simulink model "RflyUdpUltraSimpleEight_Dist"  (R2022a)
settings: Solver=FixedStepDiscrete  StartTime=0.0  StopTime=inf  FixedStep=1/30  RelTol=1e-3  EnableMultiTasking=on
PreLoadFcn:
  | filepath  = fileparts(get_param(bdroot, 'FileName'))
  | cd(filepath);
undefined symbols (not defined in the file): Busy, Wait
libraries: aerolibanimutils x1
(part 1 of 2)
settings Model: Creator=dream  LastModifiedBy=23790
settings SolverCC: AlgebraicLoopSolver=TrustRegion
settings DataIOCC: SaveFormat=Array  SignalLoggingSaveFormat=ModelDataLogs  ReturnWorkspaceOutputs=off
settings OptimizationCC: BlockReduction=off  BooleanDataType=off  ZeroExternalMemoryAtStartup=off  ZeroInternalMemoryAtStartup=off
settings DebuggingCC: SaveWithParameterizedLinksMsg=none  UnderspecifiedInitializationDetection=Classic  MergeDetectMultiDrivingBlocksExec=none  SignalResolutionControl=TryResolveAllWithWarning  MultiTaskDSMMsg=warning  MultiTaskCondExecSysMsg=none  UnconnectedInputMsg=warning  UnconnectedOutputMsg=warning  UnconnectedLineMsg=warning  SFMachineParentedDataDiag=warning  ArithmeticOperatorsInVariantConditions=warning
settings HardwareCC: TargetBitPerPointer=64  TargetBitPerSizeT=64  TargetBitPerPtrDiffT=64  TargetLongLongMode=on  TargetIntDivRoundTo=Zero  TargetEndianess=LittleEndian  TargetWordSize=64  TargetHWDeviceType=MATLAB Host  ProdEqTarget=off
settings ModelReferenceCC: PropagateSignalLabelsOutOfModel=off
settings SFSimCC: SimUseLocalCustomCode=off  CustomCodeUndefinedFunction=UseInterfaceOnly  SimTargetLang=C++
settings RTWCC: PackageGeneratedCodeAndArtifacts=on  PackageName=RflyUdpExe  RTWUseLocalCustomCode=off  BuildConfiguration=Faster Runs  TargetLang=C++
settings GRTTargetCC: TargetLangStandard=C++03 (ISO)  CodeInterfacePackaging=C++ class  MultiInstanceErrorCode=None

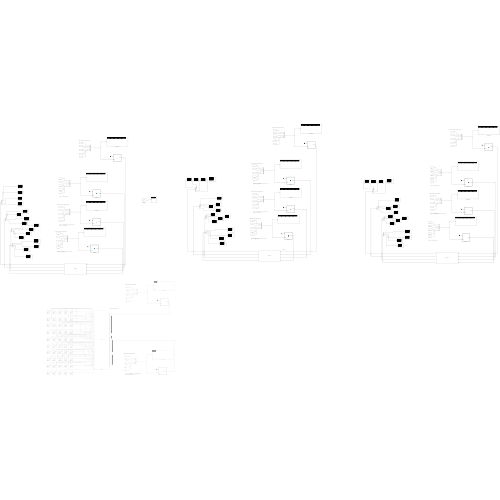
[thumbnail: Simulink's stored preview of the top-level diagram]
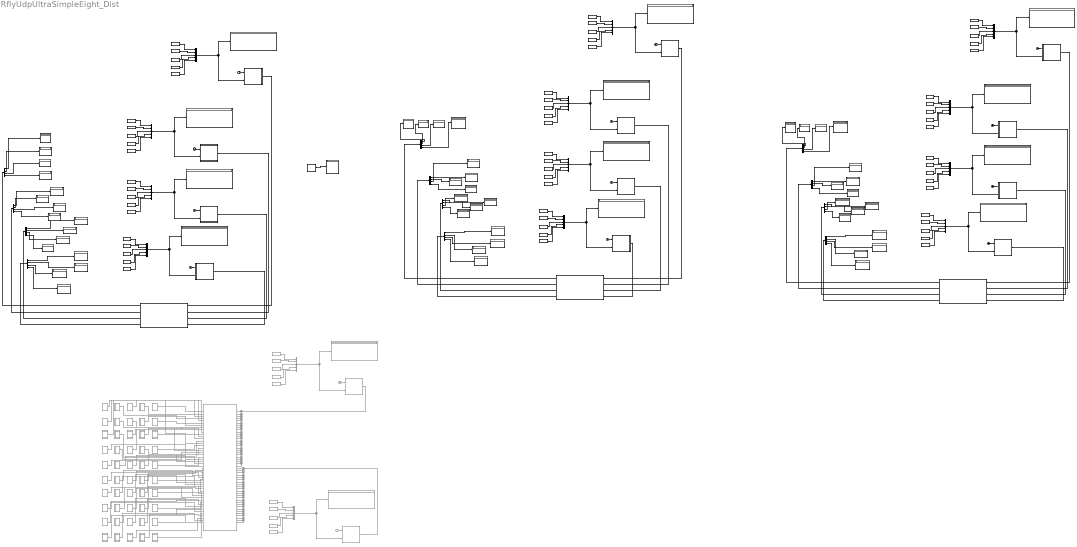
== system RflyUdpUltraSimpleEight_Dist ==
  note: 飞机状态反馈
  note: 0: Earth Vel; 1:Body Vel; 2: Earth Pos; 3:Body Pos
  note: 0: Earth Vel; 1:Body Vel; 2: Earth Pos; 3:Body Pos
  note: 这里展示了发送一条flag为2的消息，对应 地球坐标系下的位置指令
      | 发送本指令时，固定翼会飞到预设的点
  note: 这里展示了发送一条flag为2的消息，对应 地球坐标系下的位置指令
      | 发送本指令时，固定翼会飞到预设的点
  note: 0: Earth Vel; 1:Body Vel; 2: Earth Pos; 3:Body Pos
  note: 0: Earth Vel; 1:Body Vel; 2: Earth Pos; 3:Body Pos
  note: 这里展示了发送一条flag为2的消息，对应 地球坐标系下的位置指令
      | 发送本指令时，固定翼会飞到预设的点
  note: 这里展示了发送一条flag为2的消息，对应 地球坐标系下的位置指令
      | 发送本指令时，固定翼会飞到预设的点
  note: 0: Earth Vel; 1:Body Vel; 2: Earth Pos; 3:Body Pos
  note: 这里展示了发送一条flag为2的消息，对应 地球坐标系下的位置指令
      | 发送本指令时，固定翼会飞到预设的点
  note: 0: Earth Vel; 1:Body Vel; 2: Earth Pos; 3:Body Pos
  note: 0: Earth Vel; 1:Body Vel; 2: Earth Pos; 3:Body Pos
  note: 0: Earth Vel; 1:Body Vel; 2: Earth Pos; 3:Body Pos
  note: 这里展示了发送一条flag为2的消息，对应 地球坐标系下的位置指令
      | 发送本指令时，固定翼会飞到预设的点
  note: 这里展示了发送一条flag为2的消息，对应 地球坐标系下的位置指令
      | 发送本指令时，固定翼会飞到预设的点
  note: 0: Earth Vel; 1:Body Vel; 2: Earth Pos; 3:Body Pos
  note: 0: Earth Vel; 1:Body Vel; 2: Earth Pos; 3:Body Pos
  note: 这里展示了发送一条flag为2的消息，对应 地球坐标系下的位置指令
      | 发送本指令时，固定翼会飞到预设的点
  note: 飞机状态反馈
  note: 0: Earth Vel; 1:Body Vel; 2: Earth Pos; 3:Body Pos
  note: 这里展示了发送一条flag为2的消息，对应 地球坐标系下的位置指令
      | 发送本指令时，固定翼会飞到预设的点
  note: 这里展示了发送一条flag为2的消息，对应 地球坐标系下的位置指令
      | 发送本指令时，固定翼会飞到预设的点
  note: 0: Earth Vel; 1:Body Vel; 2: Earth Pos; 3:Body Pos
  note: 飞机状态反馈
  note: 0: Earth Vel; 1:Body Vel; 2: Earth Pos; 3:Body Pos
  note: 这里展示了发送一条flag为2的消息，对应 地球坐标系下的位置指令
      | 发送本指令时，固定翼会飞到预设的点
  note: 0: Earth Vel; 1:Body Vel; 2: Earth Pos; 3:Body Pos
  10号飞机状态反馈 : Subsystem  Commented=on
  10号飞机状态反馈1 : Subsystem  Commented=on
  10号飞机状态反馈2 : Subsystem  Commented=on
  10号飞机状态反馈3 : Subsystem  Commented=on
  10号飞机状态反馈4 : Subsystem  Commented=on
  1号飞机状态反馈 : Subsystem  Commented=on
  1号飞机状态反馈1 : Subsystem  Commented=on
  1号飞机状态反馈2 : Subsystem  Commented=on
  1号飞机状态反馈3 : Subsystem  Commented=on
  1号飞机状态反馈4 : Subsystem  Commented=on
  2号飞机状态反馈 : Subsystem  Commented=on
  2号飞机状态反馈1 : Subsystem  Commented=on
  2号飞机状态反馈2 : Subsystem  Commented=on
  2号飞机状态反馈3 : Subsystem  Commented=on
  2号飞机状态反馈4 : Subsystem  Commented=on
  3号飞机状态反馈 : Subsystem  Commented=on
  3号飞机状态反馈1 : Subsystem  Commented=on
  3号飞机状态反馈2 : Subsystem  Commented=on
  3号飞机状态反馈3 : Subsystem  Commented=on
  3号飞机状态反馈4 : Subsystem  Commented=on
  4号飞机状态反馈 : Subsystem  Commented=on
  4号飞机状态反馈1 : Subsystem  Commented=on
  4号飞机状态反馈2 : Subsystem  Commented=on
  4号飞机状态反馈3 : Subsystem  Commented=on
  4号飞机状态反馈4 : Subsystem  Commented=on
  5号飞机状态反馈 : Subsystem  Commented=on
  5号飞机状态反馈1 : Subsystem  Commented=on
  5号飞机状态反馈2 : Subsystem  Commented=on
  5号飞机状态反馈3 : Subsystem  Commented=on
  5号飞机状态反馈4 : Subsystem  Commented=on
  6号飞机状态反馈 : Subsystem  Commented=on
  6号飞机状态反馈1 : Subsystem  Commented=on
  6号飞机状态反馈2 : Subsystem  Commented=on
  6号飞机状态反馈3 : Subsystem  Commented=on
  6号飞机状态反馈4 : Subsystem  Commented=on
  7号飞机状态反馈 : Subsystem  Commented=on
  7号飞机状态反馈1 : Subsystem  Commented=on
  7号飞机状态反馈2 : Subsystem  Commented=on
  7号飞机状态反馈3 : Subsystem  Commented=on
  7号飞机状态反馈4 : Subsystem  Commented=on
  8号飞机状态反馈 : Subsystem  Commented=on
  8号飞机状态反馈1 : Subsystem  Commented=on
  8号飞机状态反馈2 : Subsystem  Commented=on
  8号飞机状态反馈3 : Subsystem  Commented=on
  8号飞机状态反馈4 : Subsystem  Commented=on
  9号飞机状态反馈 : Subsystem  Commented=on
  9号飞机状态反馈1 : Subsystem  Commented=on
  9号飞机状态反馈2 : Subsystem  Commented=on
  9号飞机状态反馈3 : Subsystem  Commented=on
  9号飞机状态反馈4 : Subsystem  Commented=on
  Clock : Clock  Commented=on
  Clock1 : Clock  Commented=on
  Clock{2..13} (12 alike) : Clock
  Commander : MATLAB Function  Commented=on  TreatAsAtomicUnit=on
  Commander1 : MATLAB Function  Commented=on  TreatAsAtomicUnit=on
  Commander10 : MATLAB Function  TreatAsAtomicUnit=on
  Commander11 : MATLAB Function  TreatAsAtomicUnit=on
  Commander12 : MATLAB Function  TreatAsAtomicUnit=on
  Commander13 : MATLAB Function  TreatAsAtomicUnit=on
  Commander2 : MATLAB Function  TreatAsAtomicUnit=on
  Commander3 : MATLAB Function  TreatAsAtomicUnit=on
  Commander4 : MATLAB Function  TreatAsAtomicUnit=on
  Commander5 : MATLAB Function  TreatAsAtomicUnit=on
  Commander6 : MATLAB Function  TreatAsAtomicUnit=on
  Commander7 : MATLAB Function  TreatAsAtomicUnit=on
  Commander8 : MATLAB Function  TreatAsAtomicUnit=on
  Commander9 : MATLAB Function  TreatAsAtomicUnit=on
  Demux{1..11,24} (12 alike) : Demux
  Display{,1..32,49..64} (49 alike) : Display
  Last Valid Data1 : Display  Commented=on
  Last Valid Data{2..3,5..14} (12 alike) : Display
  Last Valid Data4 : Display  Commented=on
  Mux{1..11,26} (12 alike) : Mux  Inputs=5
  Mux24 : Mux  Commented=on  Inputs=5
  Mux25 : Mux  Commented=on  Inputs=5
  PosX{,1..11} (12 alike) : Constant  Value=160
  PosX/Vel : Constant  Commented=on  Value=500
  PosX1/Vel1 : Constant  Commented=on  Value=500
  PosY{,1..11} (12 alike) : Constant  Value=-2000
  PosY/Alt : Constant  Commented=on  Value=-500
  PosY1/Yaw1 : Constant  Commented=on  Value=-500
  PosZ{,1..11} (12 alike) : Constant  Value=10/180*pi
  PosZ/Yaw : Constant  Commented=on
  PosZ1/Alt1 : Constant  Commented=on
  RflyUdpFast : S-Function  Commented=on  FunctionName=RflyUdpFast  Parameters=port,num,modeValue,T,ip  SFunctionDeploymentMode=off  EnableBusSupport=off  mask(UDP Receive){ip=192.168.31.11, port=20200, num=50, mode=UltraSimple Mode, T=1/30, modeValue=0}
      mask prompts: ip "UDP IP Address"; port "UDP Port"; num "vehicle Number"; mode "UDP Mode"; T "Sample Time"
      mask help:
      | This block receives bytes from an UDP/IP connection.
      | The first parameter is the UDP port on the first CopterSim App
      | The second parameter is the total vehicle number
      | The third parameter is the data mode. check the help button for the definition
      mask init:
      | if strcmp(mode,'FullData Mode')
      |     modeValue = 0;
      | elseif strcmp(mode,'SimpleData Mode') 
      |     modeValue = 1;
      | elseif strcmp(mode,'UltraSimple Mode') 
      |     modeValue = 2;
      | else
      |     modeValue = 0;
      | end
      mask Help:
      | UDP mode = 0 (localhost) or 1(broadcast), the 28-D output is defined as:
      | for(int i=0;i<3;i++){
      |     data[0+i]=(double)stl.gpsHome[i];
      |     data[3+i]=(double)stl.AngEular[i];
      |     data[6+i]=(double)stl.localPos[i];
      |     data[9+i]=(double)stl.localVel[i];
      |     data[12+i]=(double)stl.GpsPos[i];
      |     data[15+i]=(double)stl.GpsVel[i];
      | }
      | data[18] = (double)stl.time_boot_ms;
      | data[19] = (double)stl.copterID;
      | data[20] = (double)stl.relative_alt;
      | data[21] = (double)stl.hdg;
      | data[22] = (double)stl.satellites_visible;
      | data[23] = (double)stl.fix_type;
      | data[24] = (double)stl.resrveInit;
      | data[25] = (double)stl.pos_horiz_accuracy;
      | data[26] = (double)stl.pos_vert_accuracy;
      | data[27] = (double)stl.resrveFloat;
      | 
      | UDP mode =  2 (localhost) or 3(broadcast), 4,5 the 12-D output is defined as:
      | 
      | if(iUdpMode==2||iUdpMode==3){
      |     for(int i=0;i<3;i++){
      |         data[i]=(double)st.gpsHome[i];
      |         data[i+3]=(double)st.AngEular[i];
      |         data[i+6]=(double)st.localPos[i];
      |         data[i+9]=(double)st.localVel[i];
      |     }
      | }
      | if(iUdpMode==4||iUdpMode==5){
      |     double GpsHomePos[3];
      |     for(int i=0;i<3;i++){
      |             GpsHomePos[i] = (double)st.gpsHome[i];
      |             data[3+i]=(double)st.localPos[i];
      |             data[6+i]=(double)st.localVel[i];
      |             data[9+i]=(double)st.AngEular[i];
      |     }
      |     double PIR = 3.1415926536;
      |     data[0]=(GpsHomePos[0]*1e-7-40.1540302)/180*PIR*6362000+(double)st.localPos[0];
      |     data[1]=(GpsHomePos[1]*1e-7-116.2593683)/180*PIR*6362000+(double)st.localPos[1];
      |     data[2]=-GpsHomePos[2]*1e-3+(double)st.localPos[2];
      | }
      | 
      | The above structure is
      | struct outHILStateData{ // mavlink data forward from Pixhawk
      |     uint32_t time_boot_ms; //Timestamp of the message
      |     uint32_t copterID;     //Copter ID start from 1
      |     int32_t GpsPos[3];     //Estimated GPS position，lat&long: deg*1e7, alt: m*1e3 and up is positive
      |     int32_t GpsVel[3];     //Estimated GPS velocity, NED, m/s*1e2->cm/s
      |     int32_t gpsHome[3];     //Home GPS position, lat&long: deg*1e7, alt: m*1e3 and up is positive
      |     int32_t relative_alt;  //alt: m*1e3 and up is positive
      |     int32_t hdg;           //Course angle, NED,deg*1000, 0~360
      |     int32_t satellites_visible; //GPS Raw data, sum of satellite
      |     int32_t fix_type;     //GPS Raw data, Fixed type, 3 for fixed (good precision)
      |     int32_t resrveInit;       //Int, reserve for the future use
      |     float AngEular[3];    //Estimated Euler angle, unit: rad/s
      |     float localPos[3];    //Estimated locoal position, NED, unit: m
      |     float localVel[3];    //Estimated locoal velocity, NED, unit: m/s
      |     float pos_horiz_accuracy;   //GPS horizontal accuracy, unit: m
      |     float pos_vert_accuracy; //GPS vertical accuracy, unit: m
      |     float resrveFloat;      //float,reserve for the future use
      | }
      mask TypeOptions mode: FullData Mode | SimpleData Mode | UltraSimple Mode
  Simulation Pace1 : aerolibanimutils/Simulation Pace  SimulationPace=1  SleepMode=Busy-Wait  OutputPaceError=on  SampleTime=-1
  UDP Recv1 : S-Function  FunctionName=RflyUdpFast  Parameters=port,num,modeValue,T,ip  SFunctionDeploymentMode=off  EnableBusSupport=off  mask(UDP Receive){ip=192.168.31.253, port=20100, num=4, mode=UltraSimple Mode, T=1/30, modeValue=0}
      mask prompts: ip "UDP IP Address"; port "UDP Port"; num "vehicle Number"; mode "UDP Mode"; T "Sample Time"
      mask help:
      | This block receives bytes from an UDP/IP connection.
      | The first parameter is the UDP port on the first CopterSim App
      | The second parameter is the total vehicle number
      | The third parameter is the data mode. check the help button for the definition
      mask init:
      | if strcmp(mode,'FullData Mode')
      |     modeValue = 0;
      | elseif strcmp(mode,'SimpleData Mode') 
      |     modeValue = 1;
      | elseif strcmp(mode,'UltraSimple Mode') 
      |     modeValue = 2;
      | else
      |     modeValue = 0;
      | end
      mask Help:
      | UDP mode = 0 (localhost) or 1(broadcast), the 28-D output is defined as:
      | for(int i=0;i<3;i++){
      |     data[0+i]=(double)stl.gpsHome[i];
      |     data[3+i]=(double)stl.AngEular[i];
      |     data[6+i]=(double)stl.localPos[i];
      |     data[9+i]=(double)stl.localVel[i];
      |     data[12+i]=(double)stl.GpsPos[i];
      |     data[15+i]=(double)stl.GpsVel[i];
      | }
      | data[18] = (double)stl.time_boot_ms;
      | data[19] = (double)stl.copterID;
      | data[20] = (double)stl.relative_alt;
      | data[21] = (double)stl.hdg;
      | data[22] = (double)stl.satellites_visible;
      | data[23] = (double)stl.fix_type;
      | data[24] = (double)stl.resrveInit;
      | data[25] = (double)stl.pos_horiz_accuracy;
      | data[26] = (double)stl.pos_vert_accuracy;
      | data[27] = (double)stl.resrveFloat;
      | 
      | UDP mode =  2 (localhost) or 3(broadcast), 4,5 the 12-D output is defined as:
      | 
      | if(iUdpMode==2||iUdpMode==3){
      |     for(int i=0;i<3;i++){
      |         data[i]=(double)st.gpsHome[i];
      |         data[i+3]=(double)st.AngEular[i];
      |         data[i+6]=(double)st.localPos[i];
      |         data[i+9]=(double)st.localVel[i];
      |     }
      | }
      | if(iUdpMode==4||iUdpMode==5){
      |     double GpsHomePos[3];
      |     for(int i=0;i<3;i++){
      |             GpsHomePos[i] = (double)st.gpsHome[i];
      |             data[3+i]=(double)st.localPos[i];
      |             data[6+i]=(double)st.localVel[i];
      |             data[9+i]=(double)st.AngEular[i];
      |     }
      |     double PIR = 3.1415926536;
      |     data[0]=(GpsHomePos[0]*1e-7-40.1540302)/180*PIR*6362000+(double)st.localPos[0];
      |     data[1]=(GpsHomePos[1]*1e-7-116.2593683)/180*PIR*6362000+(double)st.localPos[1];
      |     data[2]=-GpsHomePos[2]*1e-3+(double)st.localPos[2];
      | }
      | 
      | The above structure is
      | struct outHILStateData{ // mavlink data forward from Pixhawk
      |     uint32_t time_boot_ms; //Timestamp of the message
      |     uint32_t copterID;     //Copter ID start from 1
      |     int32_t GpsPos[3];     //Estimated GPS position，lat&long: deg*1e7, alt: m*1e3 and up is positive
      |     int32_t GpsVel[3];     //Estimated GPS velocity, NED, m/s*1e2->cm/s
      |     int32_t gpsHome[3];     //Home GPS position, lat&long: deg*1e7, alt: m*1e3 and up is positive
      |     int32_t relative_alt;  //alt: m*1e3 and up is positive
      |     int32_t hdg;           //Course angle, NED,deg*1000, 0~360
      |     int32_t satellites_visible; //GPS Raw data, sum of satellite
      |     int32_t fix_type;     //GPS Raw data, Fixed type, 3 for fixed (good precision)
      |     int32_t resrveInit;       //Int, reserve for the future use
      |     float AngEular[3];    //Estimated Euler angle, unit: rad/s
      |     float localPos[3];    //Estimated locoal position, NED, unit: m
      |     float localVel[3];    //Estimated locoal velocity, NED, unit: m/s
      |     float pos_horiz_accuracy;   //GPS horizontal accuracy, unit: m
      |     float pos_vert_accuracy; //GPS vertical accuracy, unit: m
      |     float resrveFloat;      //float,reserve for the future use
      | }
      mask TypeOptions mode: FullData Mode | SimpleData Mode | UltraSimple Mode
  UDP Recv2 : S-Function  FunctionName=RflyUdpFast  Parameters=port,num,modeValue,T,ip  SFunctionDeploymentMode=off  EnableBusSupport=off  mask(UDP Receive){ip=192.168.31.15, port=20116, num=4, mode=UltraSimple Mode, T=1/30, modeValue=0}
      mask prompts: ip "UDP IP Address"; port "UDP Port"; num "vehicle Number"; mode "UDP Mode"; T "Sample Time"
      mask help:
      | This block receives bytes from an UDP/IP connection.
      | The first parameter is the UDP port on the first CopterSim App
      | The second parameter is the total vehicle number
      | The third parameter is the data mode. check the help button for the definition
      mask init:
      | if strcmp(mode,'FullData Mode')
      |     modeValue = 0;
      | elseif strcmp(mode,'SimpleData Mode') 
      |     modeValue = 1;
      | elseif strcmp(mode,'UltraSimple Mode') 
      |     modeValue = 2;
      | else
      |     modeValue = 0;
      | end
      mask Help:
      | UDP mode = 0 (localhost) or 1(broadcast), the 28-D output is defined as:
      | for(int i=0;i<3;i++){
      |     data[0+i]=(double)stl.gpsHome[i];
      |     data[3+i]=(double)stl.AngEular[i];
      |     data[6+i]=(double)stl.localPos[i];
      |     data[9+i]=(double)stl.localVel[i];
      |     data[12+i]=(double)stl.GpsPos[i];
      |     data[15+i]=(double)stl.GpsVel[i];
      | }
      | data[18] = (double)stl.time_boot_ms;
      | data[19] = (double)stl.copterID;
      | data[20] = (double)stl.relative_alt;
      | data[21] = (double)stl.hdg;
      | data[22] = (double)stl.satellites_visible;
      | data[23] = (double)stl.fix_type;
      | data[24] = (double)stl.resrveInit;
      | data[25] = (double)stl.pos_horiz_accuracy;
      | data[26] = (double)stl.pos_vert_accuracy;
      | data[27] = (double)stl.resrveFloat;
      | 
      | UDP mode =  2 (localhost) or 3(broadcast), 4,5 the 12-D output is defined as:
      | 
      | if(iUdpMode==2||iUdpMode==3){
      |     for(int i=0;i<3;i++){
      |         data[i]=(double)st.gpsHome[i];
      |         data[i+3]=(double)st.AngEular[i];
      |         data[i+6]=(double)st.localPos[i];
      |         data[i+9]=(double)st.localVel[i];
      |     }
      | }
      | if(iUdpMode==4||iUdpMode==5){
      |     double GpsHomePos[3];
      |     for(int i=0;i<3;i++){
      |             GpsHomePos[i] = (double)st.gpsHome[i];
      |             data[3+i]=(double)st.localPos[i];
      |             data[6+i]=(double)st.localVel[i];
      |             data[9+i]=(double)st.AngEular[i];
      |     }
      |     double PIR = 3.1415926536;
      |     data[0]=(GpsHomePos[0]*1e-7-40.1540302)/180*PIR*6362000+(double)st.localPos[0];
      |     data[1]=(GpsHomePos[1]*1e-7-116.2593683)/180*PIR*6362000+(double)st.localPos[1];
      |     data[2]=-GpsHomePos[2]*1e-3+(double)st.localPos[2];
      | }
      | 
      | The above structure is
      | struct outHILStateData{ // mavlink data forward from Pixhawk
      |     uint32_t time_boot_ms; //Timestamp of the message
      |     uint32_t copterID;     //Copter ID start from 1
      |     int32_t GpsPos[3];     //Estimated GPS position，lat&long: deg*1e7, alt: m*1e3 and up is positive
      |     int32_t GpsVel[3];     //Estimated GPS velocity, NED, m/s*1e2->cm/s
      |     int32_t gpsHome[3];     //Home GPS position, lat&long: deg*1e7, alt: m*1e3 and up is positive
      |     int32_t relative_alt;  //alt: m*1e3 and up is positive
      |     int32_t hdg;           //Course angle, NED,deg*1000, 0~360
      |     int32_t satellites_visible; //GPS Raw data, sum of satellite
      |     int32_t fix_type;     //GPS Raw data, Fixed type, 3 for fixed (good precision)
      |     int32_t resrveInit;       //Int, reserve for the future use
      |     float AngEular[3];    //Estimated Euler angle, unit: rad/s
      |     float localPos[3];    //Estimated locoal position, NED, unit: m
      |     float localVel[3];    //Estimated locoal velocity, NED, unit: m/s
      |     float pos_horiz_accuracy;   //GPS horizontal accuracy, unit: m
      |     float pos_vert_accuracy; //GPS vertical accuracy, unit: m
      |     float resrveFloat;      //float,reserve for the future use
      | }
      mask TypeOptions mode: FullData Mode | SimpleData Mode | UltraSimple Mode
  UDP Recv4 : S-Function  FunctionName=RflyUdpFast  Parameters=port,num,modeValue,T,ip  SFunctionDeploymentMode=off  EnableBusSupport=off  mask(UDP Receive){ip=192.168.31.13, port=20108, num=4, mode=UltraSimple Mode, T=1/30, modeValue=0}
      mask prompts: ip "UDP IP Address"; port "UDP Port"; num "vehicle Number"; mode "UDP Mode"; T "Sample Time"
      mask help:
      | This block receives bytes from an UDP/IP connection.
      | The first parameter is the UDP port on the first CopterSim App
      | The second parameter is the total vehicle number
      | The third parameter is the data mode. check the help button for the definition
      mask init:
      | if strcmp(mode,'FullData Mode')
      |     modeValue = 0;
      | elseif strcmp(mode,'SimpleData Mode') 
      |     modeValue = 1;
      | elseif strcmp(mode,'UltraSimple Mode') 
      |     modeValue = 2;
      | else
      |     modeValue = 0;
      | end
      mask Help:
      | UDP mode = 0 (localhost) or 1(broadcast), the 28-D output is defined as:
      | for(int i=0;i<3;i++){
      |     data[0+i]=(double)stl.gpsHome[i];
      |     data[3+i]=(double)stl.AngEular[i];
      |     data[6+i]=(double)stl.localPos[i];
      |     data[9+i]=(double)stl.localVel[i];
      |     data[12+i]=(double)stl.GpsPos[i];
      |     data[15+i]=(double)stl.GpsVel[i];
      | }
      | data[18] = (double)stl.time_boot_ms;
      | data[19] = (double)stl.copterID;
      | data[20] = (double)stl.relative_alt;
      | data[21] = (double)stl.hdg;
      | data[22] = (double)stl.satellites_visible;
      | data[23] = (double)stl.fix_type;
      | data[24] = (double)stl.resrveInit;
      | data[25] = (double)stl.pos_horiz_accuracy;
      | data[26] = (double)stl.pos_vert_accuracy;
      | data[27] = (double)stl.resrveFloat;
      | 
      | UDP mode =  2 (localhost) or 3(broadcast), 4,5 the 12-D output is defined as:
      | 
      | if(iUdpMode==2||iUdpMode==3){
      |     for(int i=0;i<3;i++){
      |         data[i]=(double)st.gpsHome[i];
      |         data[i+3]=(double)st.AngEular[i];
      |         data[i+6]=(double)st.localPos[i];
      |         data[i+9]=(double)st.localVel[i];
      |     }
      | }
      | if(iUdpMode==4||iUdpMode==5){
      |     double GpsHomePos[3];
      |     for(int i=0;i<3;i++){
      |             GpsHomePos[i] = (double)st.gpsHome[i];
      |             data[3+i]=(double)st.localPos[i];
      |             data[6+i]=(double)st.localVel[i];
      |             data[9+i]=(double)st.AngEular[i];
      |     }
      |     double PIR = 3.1415926536;
      |     data[0]=(GpsHomePos[0]*1e-7-40.1540302)/180*PIR*6362000+(double)st.localPos[0];
      |     data[1]=(GpsHomePos[1]*1e-7-116.2593683)/180*PIR*6362000+(double)st.localPos[1];
      |     data[2]=-GpsHomePos[2]*1e-3+(double)st.localPos[2];
      | }
      | 
      | The above structure is
      | struct outHILStateData{ // mavlink data forward from Pixhawk
      |     uint32_t time_boot_ms; //Timestamp of the message
      |     uint32_t copterID;     //Copter ID start from 1
      |     int32_t GpsPos[3];     //Estimated GPS position，lat&long: deg*1e7, alt: m*1e3 and up is positive
      |     int32_t GpsVel[3];     //Estimated GPS velocity, NED, m/s*1e2->cm/s
      |     int32_t gpsHome[3];     //Home GPS position, lat&long: deg*1e7, alt: m*1e3 and up is positive
      |     int32_t relative_alt;  //alt: m*1e3 and up is positive
      |     int32_t hdg;           //Course angle, NED,deg*1000, 0~360
      |     int32_t satellites_visible; //GPS Raw data, sum of satellite
      |     int32_t fix_type;     //GPS Raw data, Fixed type, 3 for fixed (good precision)
      |     int32_t resrveInit;       //Int, reserve for the future use
      |     float AngEular[3];    //Estimated Euler angle, unit: rad/s
      |     float localPos[3];    //Estimated locoal position, NED, unit: m
      |     float localVel[3];    //Estimated locoal velocity, NED, unit: m/s
      |     float pos_horiz_accuracy;   //GPS horizontal accuracy, unit: m
      |     float pos_vert_accuracy; //GPS vertical accuracy, unit: m
      |     float resrveFloat;      //float,reserve for the future use
      | }
      mask TypeOptions mode: FullData Mode | SimpleData Mode | UltraSimple Mode
  flag : Constant  Commented=on  Value=13
  flag1 : Constant  Commented=on  Value=13
  flag{2..13} (12 alike) : Constant  Value=13
  yaw : Constant  Commented=on  Value=0
  yaw1 : Constant  Commented=on  Value=0
  yaw{2..13} (12 alike) : Constant  Value=0
  wires:
  UDP Recv1/1 -> Demux4/1
  Simulation Pace1/1 -> Display/1
  Demux4/1 -> Display1/1
  Demux4/3 -> Display3/1
  Demux4/4 -> Display4/1
  Demux5/4 -> Display8/1
  Demux5/3 -> Display7/1
  Demux5/1 -> Display5/1
  Demux6/4 -> Display12/1
  Demux6/3 -> Display11/1
  Demux6/1 -> Display9/1
  UDP Recv1/2 -> Demux5/1
  UDP Recv1/3 -> Demux6/1
  Demux4/2 -> Display2/1
  Demux5/2 -> Display6/1
  Demux6/2 -> Display10/1
  Demux7/2 -> Display14/1
  Demux7/4 -> Display16/1
  UDP Recv1/4 -> Demux7/1
  Demux7/1 -> Display13/1
  Demux7/3 -> Display15/1
  RflyUdpFast/44 -> 4号飞机状态反馈4/1(In1)
  RflyUdpFast/9 -> 9号飞机状态反馈/1(In1)
  RflyUdpFast/48 -> 8号飞机状态反馈4/1(In1)
  Commander/1(outCMDs) -> RflyUdpFast/5, RflyUdpFast/6, RflyUdpFast/7, RflyUdpFast/8, RflyUdpFast/9, RflyUdpFast/10, RflyUdpFast/11, RflyUdpFast/12, RflyUdpFast/13, RflyUdpFast/14, RflyUdpFast/15, RflyUdpFast/16, RflyUdpFast/17, RflyUdpFast/18, RflyUdpFast/19, RflyUdpFast/20, RflyUdpFast/21, RflyUdpFast/22, RflyUdpFast/23, RflyUdpFast/24, RflyUdpFast/25, RflyUdpFast/4, RflyUdpFast/3, RflyUdpFast/2, RflyUdpFast/1
  RflyUdpFast/22 -> 2号飞机状态反馈2/1(In1)
  RflyUdpFast/27 -> 7号飞机状态反馈2/1(In1)
  RflyUdpFast/49 -> 9号飞机状态反馈4/1(In1)
  RflyUdpFast/40 -> 10号飞机状态反馈3/1(In1)
  RflyUdpFast/45 -> 5号飞机状态反馈4/1(In1)
  RflyUdpFast/18 -> 8号飞机状态反馈1/1(In1)
  RflyUdpFast/37 -> 7号飞机状态反馈3/1(In1)
  RflyUdpFast/25 -> 5号飞机状态反馈2/1(In1)
  Commander1/1(outCMDs) -> RflyUdpFast/50, RflyUdpFast/49, RflyUdpFast/48, RflyUdpFast/47, RflyUdpFast/46, RflyUdpFast/45, RflyUdpFast/44, RflyUdpFast/43, RflyUdpFast/42, RflyUdpFast/41, RflyUdpFast/40, RflyUdpFast/39, RflyUdpFast/38, RflyUdpFast/37, RflyUdpFast/36, RflyUdpFast/35, RflyUdpFast/34, RflyUdpFast/33, RflyUdpFast/32, RflyUdpFast/31, RflyUdpFast/30, RflyUdpFast/29, RflyUdpFast/28, RflyUdpFast/27, RflyUdpFast/26
  RflyUdpFast/7 -> 7号飞机状态反馈/1(In1)
  RflyUdpFast/50 -> 10号飞机状态反馈4/1(In1)
  RflyUdpFast/42 -> 2号飞机状态反馈4/1(In1)
  RflyUdpFast/3 -> 3号飞机状态反馈/1(In1)
  RflyUdpFast/39 -> 9号飞机状态反馈3/1(In1)
  yaw/1 -> Mux24/5
  RflyUdpFast/21 -> 1号飞机状态反馈2/1(In1)
  RflyUdpFast/35 -> 5号飞机状态反馈3/1(In1)
  RflyUdpFast/6 -> 6号飞机状态反馈/1(In1)
  RflyUdpFast/33 -> 3号飞机状态反馈3/1(In1)
  RflyUdpFast/34 -> 4号飞机状态反馈3/1(In1)
  RflyUdpFast/24 -> 4号飞机状态反馈2/1(In1)
  RflyUdpFast/11 -> 1号飞机状态反馈1/1(In1)
  RflyUdpFast/12 -> 2号飞机状态反馈1/1(In1)
  flag/1 -> Mux24/1
  RflyUdpFast/23 -> 3号飞机状态反馈2/1(In1)
  PosY/Alt/1 -> Mux24/3
  RflyUdpFast/47 -> 7号飞机状态反馈4/1(In1)
  RflyUdpFast/31 -> 1号飞机状态反馈3/1(In1)
  Clock1/1 -> Commander1/1(t)
  RflyUdpFast/8 -> 8号飞机状态反馈/1(In1)
  RflyUdpFast/43 -> 3号飞机状态反馈4/1(In1)
  RflyUdpFast/16 -> 6号飞机状态反馈1/1(In1)
  RflyUdpFast/29 -> 9号飞机状态反馈2/1(In1)
  RflyUdpFast/30 -> 10号飞机状态反馈2/1(In1)
  Mux25/1 -> Last Valid Data1/1, Commander1/2(inCMDs)
  Clock/1 -> Commander/1(t)
  PosX/Vel/1 -> Mux24/2
  RflyUdpFast/20 -> 10号飞机状态反馈1/1(In1)
  RflyUdpFast/19 -> 9号飞机状态反馈1/1(In1)
  RflyUdpFast/15 -> 5号飞机状态反馈1/1(In1)
  RflyUdpFast/26 -> 6号飞机状态反馈2/1(In1)
  PosY1/Yaw1/1 -> Mux25/3
  RflyUdpFast/4 -> 4号飞机状态反馈/1(In1)
  RflyUdpFast/36 -> 6号飞机状态反馈3/1(In1)
  PosZ/Yaw/1 -> Mux24/4
  RflyUdpFast/17 -> 7号飞机状态反馈1/1(In1)
  PosX1/Vel1/1 -> Mux25/2
  RflyUdpFast/5 -> 5号飞机状态反馈/1(In1)
  RflyUdpFast/38 -> 8号飞机状态反馈3/1(In1)
  yaw1/1 -> Mux25/5
  RflyUdpFast/10 -> 10号飞机状态反馈/1(In1)
  RflyUdpFast/46 -> 6号飞机状态反馈4/1(In1)
  RflyUdpFast/41 -> 1号飞机状态反馈4/1(In1)
  RflyUdpFast/13 -> 3号飞机状态反馈1/1(In1)
  RflyUdpFast/1 -> 1号飞机状态反馈/1(In1)
  RflyUdpFast/32 -> 2号飞机状态反馈3/1(In1)
  RflyUdpFast/14 -> 4号飞机状态反馈1/1(In1)
  flag1/1 -> Mux25/1
  RflyUdpFast/2 -> 2号飞机状态反馈/1(In1)
  RflyUdpFast/28 -> 8号飞机状态反馈2/1(In1)
  Mux24/1 -> Last Valid Data4/1, Commander/2(inCMDs)
  PosZ1/Alt1/1 -> Mux25/4
  yaw2/1 -> Mux26/5
  Mux26/1 -> Last Valid Data2/1, Commander2/2(inCMDs)
  PosY/1 -> Mux26/3
  Clock2/1 -> Commander2/1(t)
  flag2/1 -> Mux26/1
  PosZ/1 -> Mux26/4
  PosX/1 -> Mux26/2
  Commander2/1(outCMDs) -> UDP Recv1/1
  Clock3/1 -> Commander3/1(t)
  yaw3/1 -> Mux2/5
  PosX1/1 -> Mux2/2
  flag3/1 -> Mux2/1
  Commander3/1(outCMDs) -> UDP Recv1/2
  PosY1/1 -> Mux2/3
  Mux2/1 -> Last Valid Data3/1, Commander3/2(inCMDs)
  PosZ1/1 -> Mux2/4
  PosX2/1 -> Mux3/2
  PosY2/1 -> Mux3/3
  Commander4/1(outCMDs) -> UDP Recv1/3
  flag4/1 -> Mux3/1
  Mux3/1 -> Commander4/2(inCMDs), Last Valid Data5/1
  yaw4/1 -> Mux3/5
  Clock4/1 -> Commander4/1(t)
  PosZ2/1 -> Mux3/4
  PosY3/1 -> Mux4/3
  Clock5/1 -> Commander5/1(t)
  PosZ3/1 -> Mux4/4
  Mux4/1 -> Last Valid Data6/1, Commander5/2(inCMDs)
  Commander5/1(outCMDs) -> UDP Recv1/4
  yaw5/1 -> Mux4/5
  flag5/1 -> Mux4/1
  PosX3/1 -> Mux4/2
  Commander9/1(outCMDs) -> UDP Recv4/4
  PosX7/1 -> Mux7/2
  PosZ5/1 -> Mux1/4
  PosY5/1 -> Mux1/3
  Mux1/1 -> Last Valid Data8/1, Commander7/2(inCMDs)
  PosX5/1 -> Mux1/2
  Clock9/1 -> Commander9/1(t)
  PosY4/1 -> Mux5/3
  Commander6/1(outCMDs) -> UDP Recv4/1
  PosZ4/1 -> Mux5/4
  flag6/1 -> Mux5/1
  Commander8/1(outCMDs) -> UDP Recv4/3
  PosX4/1 -> Mux5/2
  yaw8/1 -> Mux6/5
  Clock6/1 -> Commander6/1(t)
  PosY6/1 -> Mux6/3
  PosX6/1 -> Mux6/2
  flag8/1 -> Mux6/1
  Demux24/3 -> Display55/1
  yaw6/1 -> Mux5/5
  UDP Recv4/3 -> Demux3/1
  Clock7/1 -> Commander7/1(t)
  yaw7/1 -> Mux1/5
  Demux3/2 -> Display50/1
  Demux3/3 -> Display51/1
  Clock8/1 -> Commander8/1(t)
  Demux24/4 -> Display56/1
  UDP Recv4/4 -> Demux24/1
  Demux2/1 -> Display60/1
  Demux2/3 -> Display62/1
  Demux24/1 -> Display53/1
  Mux5/1 -> Last Valid Data7/1, Commander6/2(inCMDs)
  Demux3/4 -> Display52/1
  Demux2/4 -> Display63/1
  Demux3/1 -> Display64/1
  PosY7/1 -> Mux7/3
  Demux1/1 -> Display49/1
  Demux1/3 -> Display58/1
  Mux6/1 -> Commander8/2(inCMDs), Last Valid Data9/1
  PosZ6/1 -> Mux6/4
  UDP Recv4/2 -> Demux2/1
  Demux1/4 -> Display59/1
  Demux2/2 -> Display61/1
  Mux7/1 -> Last Valid Data10/1, Commander9/2(inCMDs)
  PosZ7/1 -> Mux7/4
  Commander7/1(outCMDs) -> UDP Recv4/2
  flag9/1 -> Mux7/1
  Demux24/2 -> Display54/1
  yaw9/1 -> Mux7/5
  Demux1/2 -> Display57/1
  UDP Recv4/1 -> Demux1/1
  flag7/1 -> Mux1/1
  PosZ8/1 -> Mux9/4
  PosX8/1 -> Mux9/2
  yaw12/1 -> Mux10/5
  flag10/1 -> Mux9/1
  Commander10/1(outCMDs) -> UDP Recv2/1
  Mux8/1 -> Last Valid Data13/1, Commander11/2(inCMDs)
  PosX9/1 -> Mux8/2
  Clock13/1 -> Commander13/1(t)
  PosY9/1 -> Mux8/3
  Commander13/1(outCMDs) -> UDP Recv2/4
  Mux10/1 -> Commander12/2(inCMDs), Last Valid Data14/1
  PosY11/1 -> Mux11/3
  PosX11/1 -> Mux11/2
  Demux9/4 -> Display31/1
  Demux10/1 -> Display21/1
  Demux9/1 -> Display28/1
  UDP Recv2/4 -> Demux10/1
  Demux10/4 -> Display24/1
  Demux8/1 -> Display17/1
  Clock12/1 -> Commander12/1(t)
  yaw10/1 -> Mux9/5
  PosZ10/1 -> Mux10/4
  Demux10/3 -> Display23/1
  yaw11/1 -> Mux8/5
  Clock10/1 -> Commander10/1(t)
  Demux11/2 -> Display18/1
  Clock11/1 -> Commander11/1(t)
  Demux11/1 -> Display32/1
  PosX10/1 -> Mux10/2
  UDP Recv2/2 -> Demux9/1
  Demux8/4 -> Display27/1
  Mux9/1 -> Last Valid Data12/1, Commander10/2(inCMDs)
  UDP Recv2/1 -> Demux8/1
  flag12/1 -> Mux10/1
  flag13/1 -> Mux11/1
  PosZ9/1 -> Mux8/4
  Mux11/1 -> Last Valid Data11/1, Commander13/2(inCMDs)
  Demux8/3 -> Display26/1
  PosY8/1 -> Mux9/3
  Demux9/2 -> Display29/1
  Demux11/3 -> Display19/1
  yaw13/1 -> Mux11/5
  PosY10/1 -> Mux10/3
  Demux11/4 -> Display20/1
  Commander11/1(outCMDs) -> UDP Recv2/2
  Demux10/2 -> Display22/1
  flag11/1 -> Mux8/1
  Demux9/3 -> Display30/1
  Demux8/2 -> Display25/1
  PosZ11/1 -> Mux11/4
  UDP Recv2/3 -> Demux11/1
  Commander12/1(outCMDs) -> UDP Recv2/3

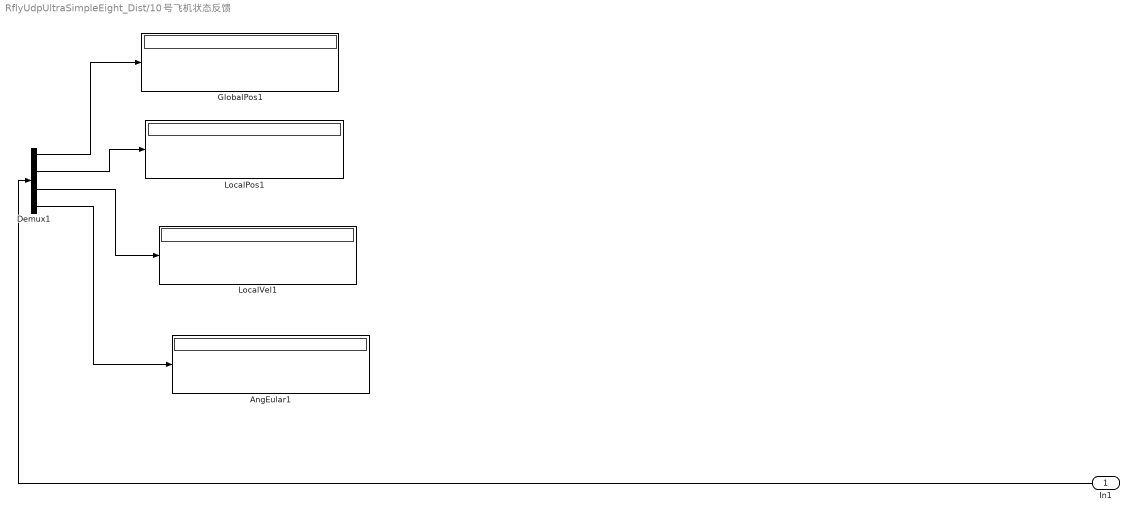
== system RflyUdpUltraSimpleEight_Dist/10号飞机状态反馈 ==
  In1 : Inport
  AngEular1 : Display
  Demux1 : Demux
  GlobalPos1 : Display
  LocalPos1 : Display
  LocalVel1 : Display
  wires:
  Demux1/2 -> LocalPos1/1
  Demux1/3 -> LocalVel1/1
  In1/1 -> Demux1/1
  Demux1/1 -> GlobalPos1/1
  Demux1/4 -> AngEular1/1

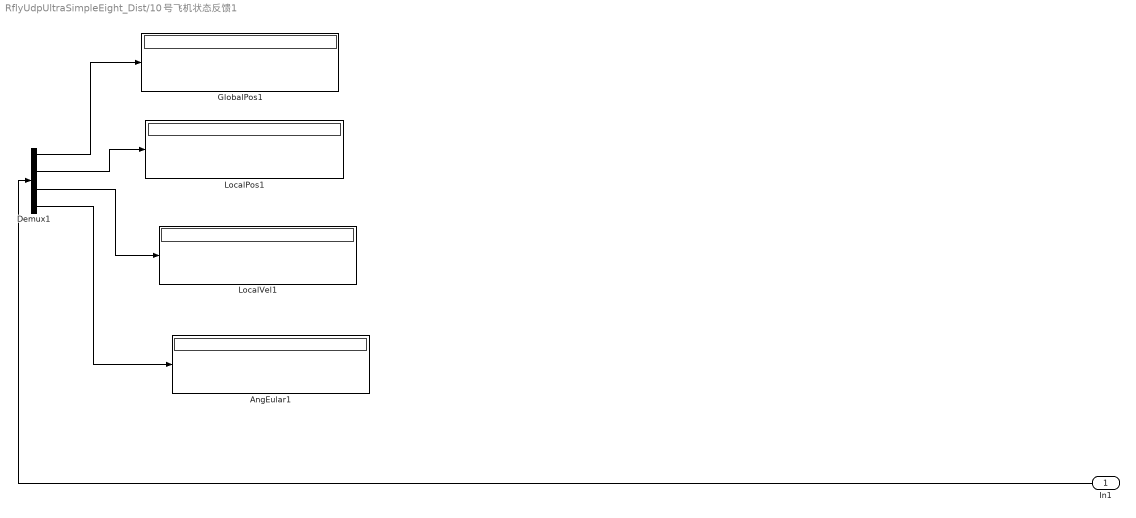
== system RflyUdpUltraSimpleEight_Dist/10号飞机状态反馈1 ==
  In1 : Inport
  AngEular1 : Display
  Demux1 : Demux
  GlobalPos1 : Display
  LocalPos1 : Display
  LocalVel1 : Display
  wires:
  Demux1/2 -> LocalPos1/1
  Demux1/3 -> LocalVel1/1
  In1/1 -> Demux1/1
  Demux1/1 -> GlobalPos1/1
  Demux1/4 -> AngEular1/1

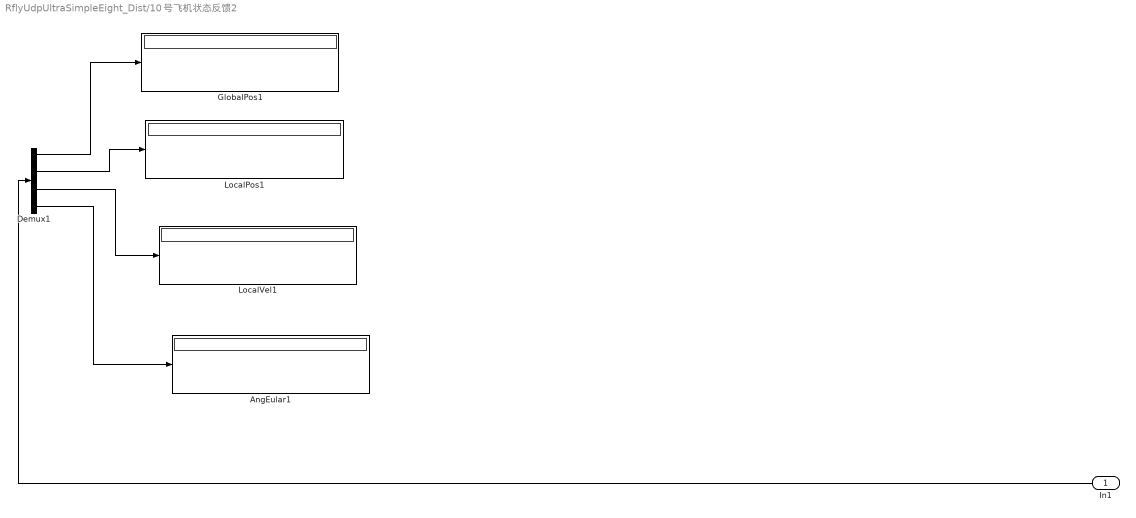
== system RflyUdpUltraSimpleEight_Dist/10号飞机状态反馈2 ==
  In1 : Inport
  AngEular1 : Display
  Demux1 : Demux
  GlobalPos1 : Display
  LocalPos1 : Display
  LocalVel1 : Display
  wires:
  Demux1/2 -> LocalPos1/1
  Demux1/3 -> LocalVel1/1
  In1/1 -> Demux1/1
  Demux1/1 -> GlobalPos1/1
  Demux1/4 -> AngEular1/1

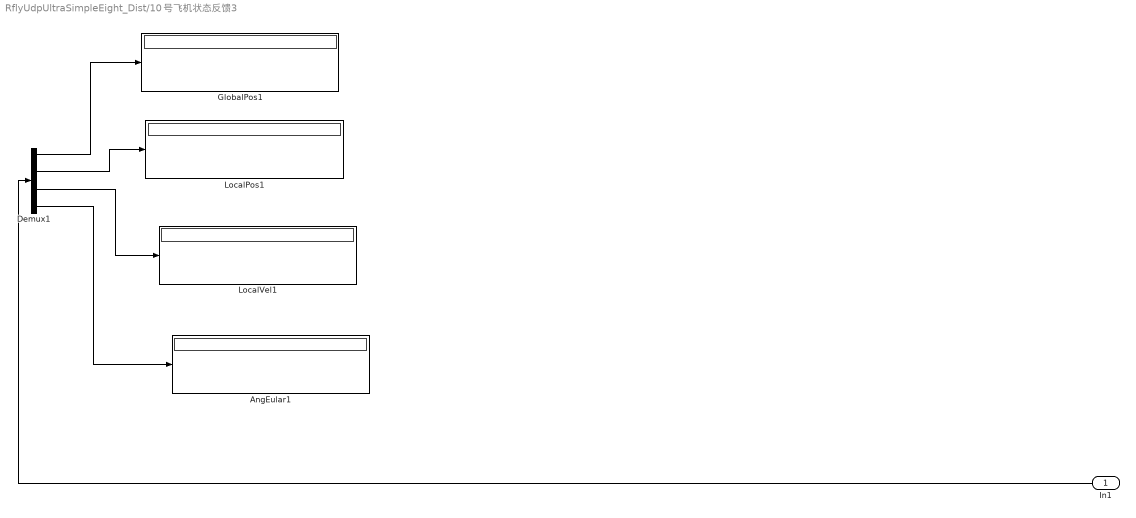
== system RflyUdpUltraSimpleEight_Dist/10号飞机状态反馈3 ==
  In1 : Inport
  AngEular1 : Display
  Demux1 : Demux
  GlobalPos1 : Display
  LocalPos1 : Display
  LocalVel1 : Display
  wires:
  Demux1/2 -> LocalPos1/1
  Demux1/3 -> LocalVel1/1
  In1/1 -> Demux1/1
  Demux1/1 -> GlobalPos1/1
  Demux1/4 -> AngEular1/1

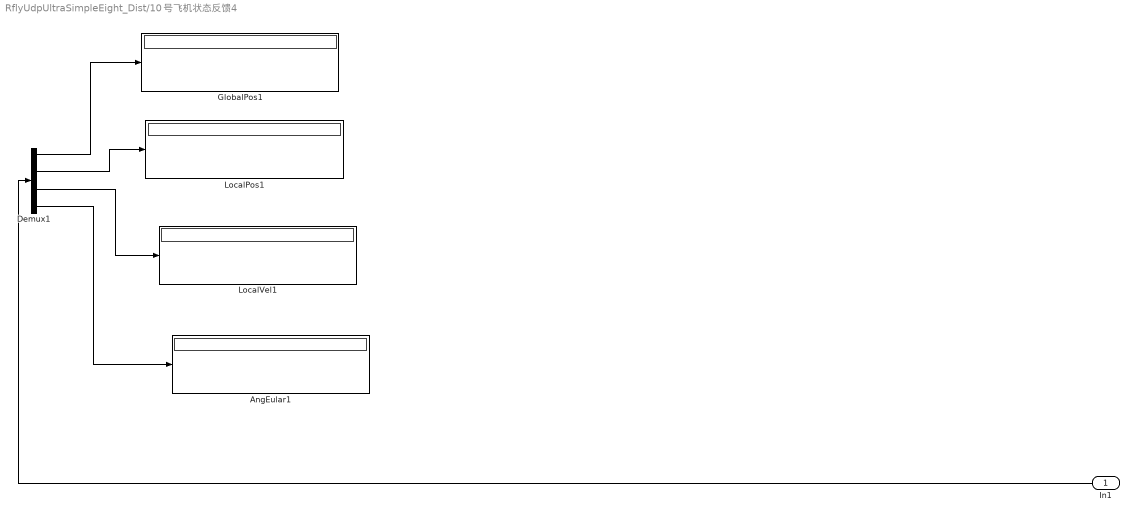
== system RflyUdpUltraSimpleEight_Dist/10号飞机状态反馈4 ==
  In1 : Inport
  AngEular1 : Display
  Demux1 : Demux
  GlobalPos1 : Display
  LocalPos1 : Display
  LocalVel1 : Display
  wires:
  Demux1/2 -> LocalPos1/1
  Demux1/3 -> LocalVel1/1
  In1/1 -> Demux1/1
  Demux1/1 -> GlobalPos1/1
  Demux1/4 -> AngEular1/1

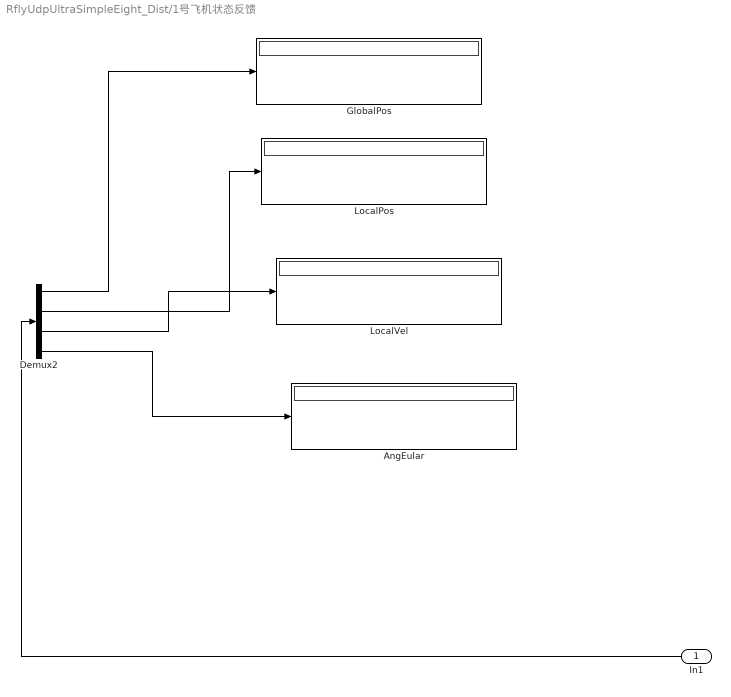
== system RflyUdpUltraSimpleEight_Dist/1号飞机状态反馈 ==
  In1 : Inport
  AngEular : Display
  Demux2 : Demux
  GlobalPos : Display
  LocalPos : Display
  LocalVel : Display
  wires:
  Demux2/4 -> AngEular/1
  Demux2/1 -> GlobalPos/1
  Demux2/2 -> LocalPos/1
  In1/1 -> Demux2/1
  Demux2/3 -> LocalVel/1

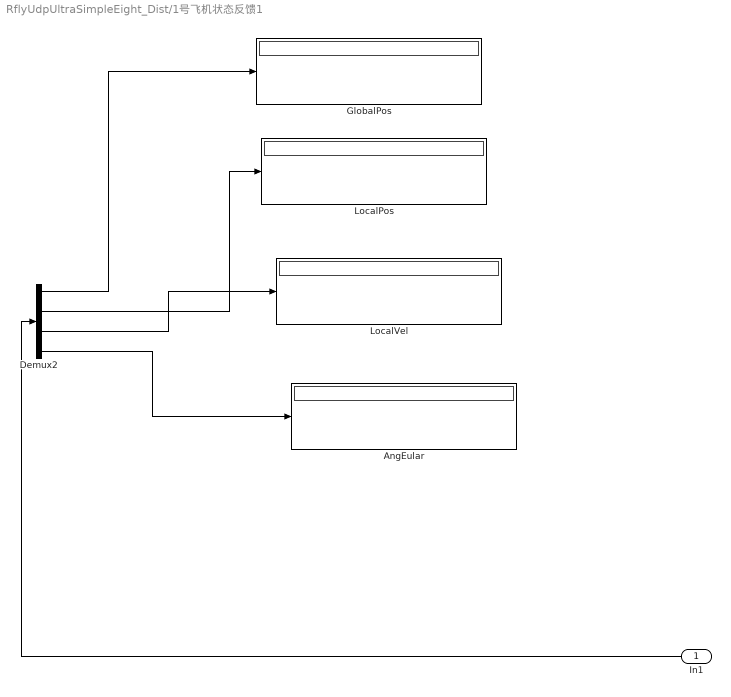
== system RflyUdpUltraSimpleEight_Dist/1号飞机状态反馈1 ==
  In1 : Inport
  AngEular : Display
  Demux2 : Demux
  GlobalPos : Display
  LocalPos : Display
  LocalVel : Display
  wires:
  Demux2/4 -> AngEular/1
  Demux2/1 -> GlobalPos/1
  Demux2/2 -> LocalPos/1
  In1/1 -> Demux2/1
  Demux2/3 -> LocalVel/1

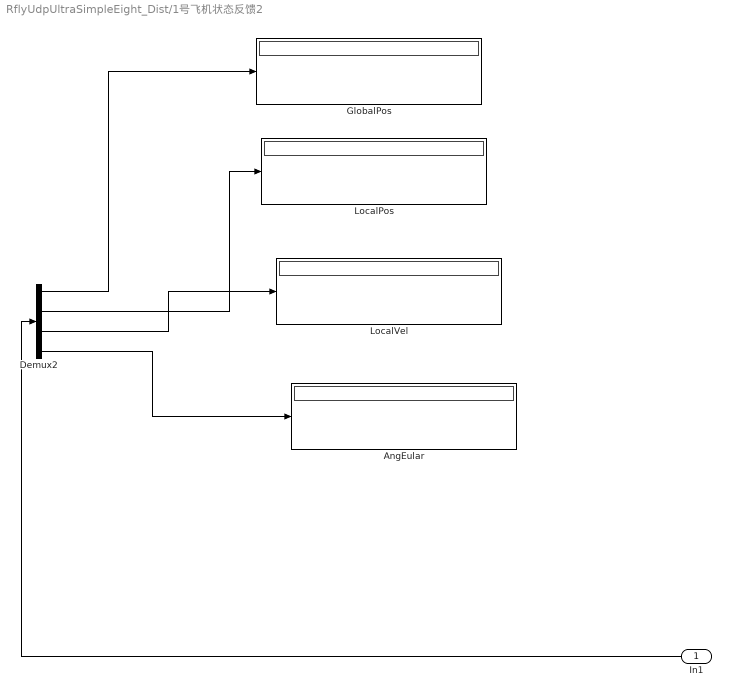
== system RflyUdpUltraSimpleEight_Dist/1号飞机状态反馈2 ==
  In1 : Inport
  AngEular : Display
  Demux2 : Demux
  GlobalPos : Display
  LocalPos : Display
  LocalVel : Display
  wires:
  Demux2/4 -> AngEular/1
  Demux2/1 -> GlobalPos/1
  Demux2/2 -> LocalPos/1
  In1/1 -> Demux2/1
  Demux2/3 -> LocalVel/1

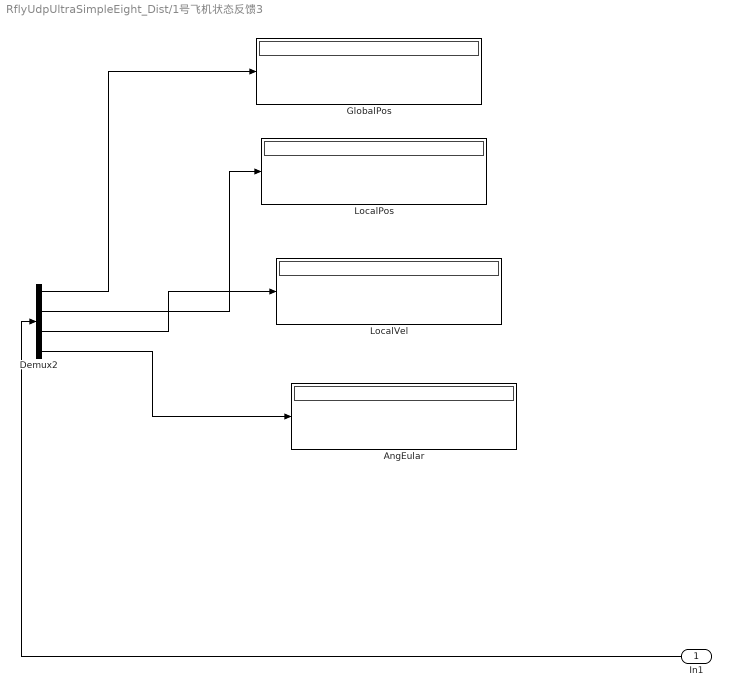
== system RflyUdpUltraSimpleEight_Dist/1号飞机状态反馈3 ==
  In1 : Inport
  AngEular : Display
  Demux2 : Demux
  GlobalPos : Display
  LocalPos : Display
  LocalVel : Display
  wires:
  Demux2/4 -> AngEular/1
  Demux2/1 -> GlobalPos/1
  Demux2/2 -> LocalPos/1
  In1/1 -> Demux2/1
  Demux2/3 -> LocalVel/1

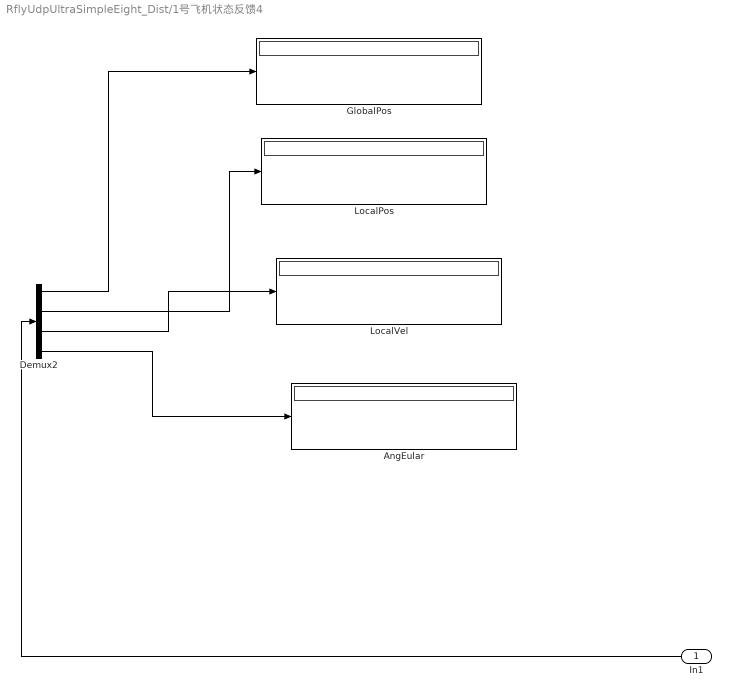
== system RflyUdpUltraSimpleEight_Dist/1号飞机状态反馈4 ==
  In1 : Inport
  AngEular : Display
  Demux2 : Demux
  GlobalPos : Display
  LocalPos : Display
  LocalVel : Display
  wires:
  Demux2/4 -> AngEular/1
  Demux2/1 -> GlobalPos/1
  Demux2/2 -> LocalPos/1
  In1/1 -> Demux2/1
  Demux2/3 -> LocalVel/1

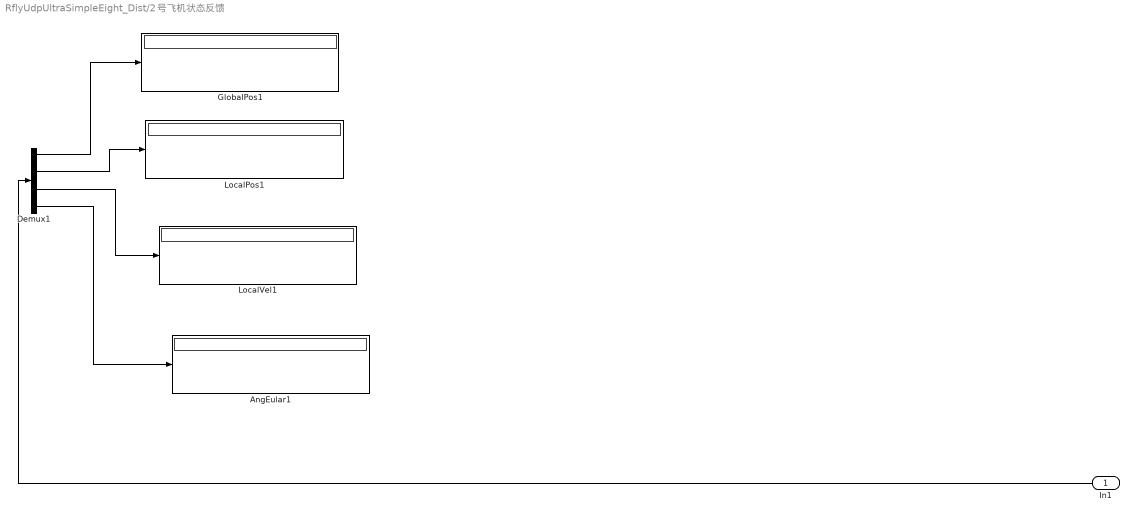
== system RflyUdpUltraSimpleEight_Dist/2号飞机状态反馈 ==
  In1 : Inport
  AngEular1 : Display
  Demux1 : Demux
  GlobalPos1 : Display
  LocalPos1 : Display
  LocalVel1 : Display
  wires:
  Demux1/2 -> LocalPos1/1
  Demux1/3 -> LocalVel1/1
  In1/1 -> Demux1/1
  Demux1/1 -> GlobalPos1/1
  Demux1/4 -> AngEular1/1

== system RflyUdpUltraSimpleEight_Dist/2号飞机状态反馈1 ==
  In1 : Inport
  AngEular1 : Display
  Demux1 : Demux
  GlobalPos1 : Display
  LocalPos1 : Display
  LocalVel1 : Display
  wires:
  Demux1/2 -> LocalPos1/1
  Demux1/3 -> LocalVel1/1
  In1/1 -> Demux1/1
  Demux1/1 -> GlobalPos1/1
  Demux1/4 -> AngEular1/1

== system RflyUdpUltraSimpleEight_Dist/2号飞机状态反馈2 ==
  In1 : Inport
  AngEular1 : Display
  Demux1 : Demux
  GlobalPos1 : Display
  LocalPos1 : Display
  LocalVel1 : Display
  wires:
  Demux1/2 -> LocalPos1/1
  Demux1/3 -> LocalVel1/1
  In1/1 -> Demux1/1
  Demux1/1 -> GlobalPos1/1
  Demux1/4 -> AngEular1/1

== system RflyUdpUltraSimpleEight_Dist/2号飞机状态反馈3 ==
  In1 : Inport
  AngEular1 : Display
  Demux1 : Demux
  GlobalPos1 : Display
  LocalPos1 : Display
  LocalVel1 : Display
  wires:
  Demux1/2 -> LocalPos1/1
  Demux1/3 -> LocalVel1/1
  In1/1 -> Demux1/1
  Demux1/1 -> GlobalPos1/1
  Demux1/4 -> AngEular1/1

== system RflyUdpUltraSimpleEight_Dist/2号飞机状态反馈4 ==
  In1 : Inport
  AngEular1 : Display
  Demux1 : Demux
  GlobalPos1 : Display
  LocalPos1 : Display
  LocalVel1 : Display
  wires:
  Demux1/2 -> LocalPos1/1
  Demux1/3 -> LocalVel1/1
  In1/1 -> Demux1/1
  Demux1/1 -> GlobalPos1/1
  Demux1/4 -> AngEular1/1

== system RflyUdpUltraSimpleEight_Dist/3号飞机状态反馈 ==
  In1 : Inport
  AngEular1 : Display
  Demux1 : Demux
  GlobalPos1 : Display
  LocalPos1 : Display
  LocalVel1 : Display
  wires:
  Demux1/2 -> LocalPos1/1
  Demux1/3 -> LocalVel1/1
  In1/1 -> Demux1/1
  Demux1/1 -> GlobalPos1/1
  Demux1/4 -> AngEular1/1

== system RflyUdpUltraSimpleEight_Dist/3号飞机状态反馈1 ==
  In1 : Inport
  AngEular1 : Display
  Demux1 : Demux
  GlobalPos1 : Display
  LocalPos1 : Display
  LocalVel1 : Display
  wires:
  Demux1/2 -> LocalPos1/1
  Demux1/3 -> LocalVel1/1
  In1/1 -> Demux1/1
  Demux1/1 -> GlobalPos1/1
  Demux1/4 -> AngEular1/1

== system RflyUdpUltraSimpleEight_Dist/3号飞机状态反馈2 ==
  In1 : Inport
  AngEular1 : Display
  Demux1 : Demux
  GlobalPos1 : Display
  LocalPos1 : Display
  LocalVel1 : Display
  wires:
  Demux1/2 -> LocalPos1/1
  Demux1/3 -> LocalVel1/1
  In1/1 -> Demux1/1
  Demux1/1 -> GlobalPos1/1
  Demux1/4 -> AngEular1/1

== system RflyUdpUltraSimpleEight_Dist/3号飞机状态反馈3 ==
  In1 : Inport
  AngEular1 : Display
  Demux1 : Demux
  GlobalPos1 : Display
  LocalPos1 : Display
  LocalVel1 : Display
  wires:
  Demux1/2 -> LocalPos1/1
  Demux1/3 -> LocalVel1/1
  In1/1 -> Demux1/1
  Demux1/1 -> GlobalPos1/1
  Demux1/4 -> AngEular1/1

== system RflyUdpUltraSimpleEight_Dist/3号飞机状态反馈4 ==
  In1 : Inport
  AngEular1 : Display
  Demux1 : Demux
  GlobalPos1 : Display
  LocalPos1 : Display
  LocalVel1 : Display
  wires:
  Demux1/2 -> LocalPos1/1
  Demux1/3 -> LocalVel1/1
  In1/1 -> Demux1/1
  Demux1/1 -> GlobalPos1/1
  Demux1/4 -> AngEular1/1

== system RflyUdpUltraSimpleEight_Dist/4号飞机状态反馈 ==
  In1 : Inport
  AngEular1 : Display
  Demux1 : Demux
  GlobalPos1 : Display
  LocalPos1 : Display
  LocalVel1 : Display
  wires:
  Demux1/2 -> LocalPos1/1
  Demux1/3 -> LocalVel1/1
  In1/1 -> Demux1/1
  Demux1/1 -> GlobalPos1/1
  Demux1/4 -> AngEular1/1

== system RflyUdpUltraSimpleEight_Dist/4号飞机状态反馈1 ==
  In1 : Inport
  AngEular1 : Display
  Demux1 : Demux
  GlobalPos1 : Display
  LocalPos1 : Display
  LocalVel1 : Display
  wires:
  Demux1/2 -> LocalPos1/1
  Demux1/3 -> LocalVel1/1
  In1/1 -> Demux1/1
  Demux1/1 -> GlobalPos1/1
  Demux1/4 -> AngEular1/1

== system RflyUdpUltraSimpleEight_Dist/4号飞机状态反馈2 ==
  In1 : Inport
  AngEular1 : Display
  Demux1 : Demux
  GlobalPos1 : Display
  LocalPos1 : Display
  LocalVel1 : Display
  wires:
  Demux1/2 -> LocalPos1/1
  Demux1/3 -> LocalVel1/1
  In1/1 -> Demux1/1
  Demux1/1 -> GlobalPos1/1
  Demux1/4 -> AngEular1/1

== system RflyUdpUltraSimpleEight_Dist/4号飞机状态反馈3 ==
  In1 : Inport
  AngEular1 : Display
  Demux1 : Demux
  GlobalPos1 : Display
  LocalPos1 : Display
  LocalVel1 : Display
  wires:
  Demux1/2 -> LocalPos1/1
  Demux1/3 -> LocalVel1/1
  In1/1 -> Demux1/1
  Demux1/1 -> GlobalPos1/1
  Demux1/4 -> AngEular1/1

== system RflyUdpUltraSimpleEight_Dist/4号飞机状态反馈4 ==
  In1 : Inport
  AngEular1 : Display
  Demux1 : Demux
  GlobalPos1 : Display
  LocalPos1 : Display
  LocalVel1 : Display
  wires:
  Demux1/2 -> LocalPos1/1
  Demux1/3 -> LocalVel1/1
  In1/1 -> Demux1/1
  Demux1/1 -> GlobalPos1/1
  Demux1/4 -> AngEular1/1

== system RflyUdpUltraSimpleEight_Dist/5号飞机状态反馈 ==
  In1 : Inport
  AngEular1 : Display
  Demux1 : Demux
  GlobalPos1 : Display
  LocalPos1 : Display
  LocalVel1 : Display
  wires:
  Demux1/2 -> LocalPos1/1
  Demux1/3 -> LocalVel1/1
  In1/1 -> Demux1/1
  Demux1/1 -> GlobalPos1/1
  Demux1/4 -> AngEular1/1

== system RflyUdpUltraSimpleEight_Dist/5号飞机状态反馈1 ==
  In1 : Inport
  AngEular1 : Display
  Demux1 : Demux
  GlobalPos1 : Display
  LocalPos1 : Display
  LocalVel1 : Display
  wires:
  Demux1/2 -> LocalPos1/1
  Demux1/3 -> LocalVel1/1
  In1/1 -> Demux1/1
  Demux1/1 -> GlobalPos1/1
  Demux1/4 -> AngEular1/1

== system RflyUdpUltraSimpleEight_Dist/5号飞机状态反馈2 ==
  In1 : Inport
  AngEular1 : Display
  Demux1 : Demux
  GlobalPos1 : Display
  LocalPos1 : Display
  LocalVel1 : Display
  wires:
  Demux1/2 -> LocalPos1/1
  Demux1/3 -> LocalVel1/1
  In1/1 -> Demux1/1
  Demux1/1 -> GlobalPos1/1
  Demux1/4 -> AngEular1/1

== system RflyUdpUltraSimpleEight_Dist/5号飞机状态反馈3 ==
  In1 : Inport
  AngEular1 : Display
  Demux1 : Demux
  GlobalPos1 : Display
  LocalPos1 : Display
  LocalVel1 : Display
  wires:
  Demux1/2 -> LocalPos1/1
  Demux1/3 -> LocalVel1/1
  In1/1 -> Demux1/1
  Demux1/1 -> GlobalPos1/1
  Demux1/4 -> AngEular1/1

== system RflyUdpUltraSimpleEight_Dist/5号飞机状态反馈4 ==
  In1 : Inport
  AngEular1 : Display
  Demux1 : Demux
  GlobalPos1 : Display
  LocalPos1 : Display
  LocalVel1 : Display
  wires:
  Demux1/2 -> LocalPos1/1
  Demux1/3 -> LocalVel1/1
  In1/1 -> Demux1/1
  Demux1/1 -> GlobalPos1/1
  Demux1/4 -> AngEular1/1

== system RflyUdpUltraSimpleEight_Dist/6号飞机状态反馈 ==
  In1 : Inport
  AngEular1 : Display
  Demux1 : Demux
  GlobalPos1 : Display
  LocalPos1 : Display
  LocalVel1 : Display
  wires:
  Demux1/2 -> LocalPos1/1
  Demux1/3 -> LocalVel1/1
  In1/1 -> Demux1/1
  Demux1/1 -> GlobalPos1/1
  Demux1/4 -> AngEular1/1

== system RflyUdpUltraSimpleEight_Dist/6号飞机状态反馈1 ==
  In1 : Inport
  AngEular1 : Display
  Demux1 : Demux
  GlobalPos1 : Display
  LocalPos1 : Display
  LocalVel1 : Display
  wires:
  Demux1/2 -> LocalPos1/1
  Demux1/3 -> LocalVel1/1
  In1/1 -> Demux1/1
  Demux1/1 -> GlobalPos1/1
  Demux1/4 -> AngEular1/1

== system RflyUdpUltraSimpleEight_Dist/6号飞机状态反馈2 ==
  In1 : Inport
  AngEular1 : Display
  Demux1 : Demux
  GlobalPos1 : Display
  LocalPos1 : Display
  LocalVel1 : Display
  wires:
  Demux1/2 -> LocalPos1/1
  Demux1/3 -> LocalVel1/1
  In1/1 -> Demux1/1
  Demux1/1 -> GlobalPos1/1
  Demux1/4 -> AngEular1/1

== system RflyUdpUltraSimpleEight_Dist/6号飞机状态反馈3 ==
  In1 : Inport
  AngEular1 : Display
  Demux1 : Demux
  GlobalPos1 : Display
  LocalPos1 : Display
  LocalVel1 : Display
  wires:
  Demux1/2 -> LocalPos1/1
  Demux1/3 -> LocalVel1/1
  In1/1 -> Demux1/1
  Demux1/1 -> GlobalPos1/1
  Demux1/4 -> AngEular1/1

== system RflyUdpUltraSimpleEight_Dist/6号飞机状态反馈4 ==
  In1 : Inport
  AngEular1 : Display
  Demux1 : Demux
  GlobalPos1 : Display
  LocalPos1 : Display
  LocalVel1 : Display
  wires:
  Demux1/2 -> LocalPos1/1
  Demux1/3 -> LocalVel1/1
  In1/1 -> Demux1/1
  Demux1/1 -> GlobalPos1/1
  Demux1/4 -> AngEular1/1

== system RflyUdpUltraSimpleEight_Dist/7号飞机状态反馈 ==
  In1 : Inport
  AngEular1 : Display
  Demux1 : Demux
  GlobalPos1 : Display
  LocalPos1 : Display
  LocalVel1 : Display
  wires:
  Demux1/2 -> LocalPos1/1
  Demux1/3 -> LocalVel1/1
  In1/1 -> Demux1/1
  Demux1/1 -> GlobalPos1/1
  Demux1/4 -> AngEular1/1

== system RflyUdpUltraSimpleEight_Dist/7号飞机状态反馈1 ==
  In1 : Inport
  AngEular1 : Display
  Demux1 : Demux
  GlobalPos1 : Display
  LocalPos1 : Display
  LocalVel1 : Display
  wires:
  Demux1/2 -> LocalPos1/1
  Demux1/3 -> LocalVel1/1
  In1/1 -> Demux1/1
  Demux1/1 -> GlobalPos1/1
  Demux1/4 -> AngEular1/1

== system RflyUdpUltraSimpleEight_Dist/7号飞机状态反馈2 ==
  In1 : Inport
  AngEular1 : Display
  Demux1 : Demux
  GlobalPos1 : Display
  LocalPos1 : Display
  LocalVel1 : Display
  wires:
  Demux1/2 -> LocalPos1/1
  Demux1/3 -> LocalVel1/1
  In1/1 -> Demux1/1
  Demux1/1 -> GlobalPos1/1
  Demux1/4 -> AngEular1/1

== system RflyUdpUltraSimpleEight_Dist/7号飞机状态反馈3 ==
  In1 : Inport
  AngEular1 : Display
  Demux1 : Demux
  GlobalPos1 : Display
  LocalPos1 : Display
  LocalVel1 : Display
  wires:
  Demux1/2 -> LocalPos1/1
  Demux1/3 -> LocalVel1/1
  In1/1 -> Demux1/1
  Demux1/1 -> GlobalPos1/1
  Demux1/4 -> AngEular1/1

== system RflyUdpUltraSimpleEight_Dist/7号飞机状态反馈4 ==
  In1 : Inport
  AngEular1 : Display
  Demux1 : Demux
  GlobalPos1 : Display
  LocalPos1 : Display
  LocalVel1 : Display
  wires:
  Demux1/2 -> LocalPos1/1
  Demux1/3 -> LocalVel1/1
  In1/1 -> Demux1/1
  Demux1/1 -> GlobalPos1/1
  Demux1/4 -> AngEular1/1

== system RflyUdpUltraSimpleEight_Dist/8号飞机状态反馈 ==
  In1 : Inport
  AngEular1 : Display
  Demux1 : Demux
  GlobalPos1 : Display
  LocalPos1 : Display
  LocalVel1 : Display
  wires:
  Demux1/2 -> LocalPos1/1
  Demux1/3 -> LocalVel1/1
  In1/1 -> Demux1/1
  Demux1/1 -> GlobalPos1/1
  Demux1/4 -> AngEular1/1

== system RflyUdpUltraSimpleEight_Dist/8号飞机状态反馈1 ==
  In1 : Inport
  AngEular1 : Display
  Demux1 : Demux
  GlobalPos1 : Display
  LocalPos1 : Display
  LocalVel1 : Display
  wires:
  Demux1/2 -> LocalPos1/1
  Demux1/3 -> LocalVel1/1
  In1/1 -> Demux1/1
  Demux1/1 -> GlobalPos1/1
  Demux1/4 -> AngEular1/1

== system RflyUdpUltraSimpleEight_Dist/8号飞机状态反馈2 ==
  In1 : Inport
  AngEular1 : Display
  Demux1 : Demux
  GlobalPos1 : Display
  LocalPos1 : Display
  LocalVel1 : Display
  wires:
  Demux1/2 -> LocalPos1/1
  Demux1/3 -> LocalVel1/1
  In1/1 -> Demux1/1
  Demux1/1 -> GlobalPos1/1
  Demux1/4 -> AngEular1/1

== system RflyUdpUltraSimpleEight_Dist/8号飞机状态反馈3 ==
  In1 : Inport
  AngEular1 : Display
  Demux1 : Demux
  GlobalPos1 : Display
  LocalPos1 : Display
  LocalVel1 : Display
  wires:
  Demux1/2 -> LocalPos1/1
  Demux1/3 -> LocalVel1/1
  In1/1 -> Demux1/1
  Demux1/1 -> GlobalPos1/1
  Demux1/4 -> AngEular1/1

== system RflyUdpUltraSimpleEight_Dist/8号飞机状态反馈4 ==
  In1 : Inport
  AngEular1 : Display
  Demux1 : Demux
  GlobalPos1 : Display
  LocalPos1 : Display
  LocalVel1 : Display
  wires:
  Demux1/2 -> LocalPos1/1
  Demux1/3 -> LocalVel1/1
  In1/1 -> Demux1/1
  Demux1/1 -> GlobalPos1/1
  Demux1/4 -> AngEular1/1

== system RflyUdpUltraSimpleEight_Dist/9号飞机状态反馈 ==
  In1 : Inport
  AngEular1 : Display
  Demux1 : Demux
  GlobalPos1 : Display
  LocalPos1 : Display
  LocalVel1 : Display
  wires:
  Demux1/2 -> LocalPos1/1
  Demux1/3 -> LocalVel1/1
  In1/1 -> Demux1/1
  Demux1/1 -> GlobalPos1/1
  Demux1/4 -> AngEular1/1

== system RflyUdpUltraSimpleEight_Dist/9号飞机状态反馈1 ==
  In1 : Inport
  AngEular1 : Display
  Demux1 : Demux
  GlobalPos1 : Display
  LocalPos1 : Display
  LocalVel1 : Display
  wires:
  Demux1/2 -> LocalPos1/1
  Demux1/3 -> LocalVel1/1
  In1/1 -> Demux1/1
  Demux1/1 -> GlobalPos1/1
  Demux1/4 -> AngEular1/1

== system RflyUdpUltraSimpleEight_Dist/9号飞机状态反馈2 ==
  In1 : Inport
  AngEular1 : Display
  Demux1 : Demux
  GlobalPos1 : Display
  LocalPos1 : Display
  LocalVel1 : Display
  wires:
  Demux1/2 -> LocalPos1/1
  Demux1/3 -> LocalVel1/1
  In1/1 -> Demux1/1
  Demux1/1 -> GlobalPos1/1
  Demux1/4 -> AngEular1/1

== system RflyUdpUltraSimpleEight_Dist/9号飞机状态反馈3 ==
  In1 : Inport
  AngEular1 : Display
  Demux1 : Demux
  GlobalPos1 : Display
  LocalPos1 : Display
  LocalVel1 : Display
  wires:
  Demux1/2 -> LocalPos1/1
  Demux1/3 -> LocalVel1/1
  In1/1 -> Demux1/1
  Demux1/1 -> GlobalPos1/1
  Demux1/4 -> AngEular1/1

== system RflyUdpUltraSimpleEight_Dist/9号飞机状态反馈4 ==
  In1 : Inport
  AngEular1 : Display
  Demux1 : Demux
  GlobalPos1 : Display
  LocalPos1 : Display
  LocalVel1 : Display
  wires:
  Demux1/2 -> LocalPos1/1
  Demux1/3 -> LocalVel1/1
  In1/1 -> Demux1/1
  Demux1/1 -> GlobalPos1/1
  Demux1/4 -> AngEular1/1

== matlab function RflyUdpUltraSimpleEight_Dist/Commander11 ==
  data: t input; inCMDs input; outCMDs output
function outCMDs  = fcn(t,inCMDs)

outCMDs=[-1;0;0;0;0]; % 默认空指令，不会发出

persistent mode;

if isempty(mode)
    mode=0;
end


% 进入1阶段，发送起飞指令
if mode==0 && t>1
    flag=11; % 这里对应本地起飞指令
    posX = 200; % x坐标
    posY=0; % y坐标
    posZ=-100;% z坐标
    outCMDs=[flag;posX;posY;posZ;0];
    mode=1;
end

% 10秒后，进入2模式
if mode==1 && t>5
    mode=2;
end


if mode==2
    outCMDs=inCMDs;
end

== matlab function RflyUdpUltraSimpleEight_Dist/Commander12 ==
  data: t input; inCMDs input; outCMDs output
function outCMDs  = fcn(t,inCMDs)

outCMDs=[-1;0;0;0;0]; % 默认空指令，不会发出

persistent mode;

if isempty(mode)
    mode=0;
end


% 进入1阶段，发送起飞指令
if mode==0 && t>1
    flag=11; % 这里对应本地起飞指令
    posX = 200; % x坐标
    posY=0; % y坐标
    posZ=-100;% z坐标
    outCMDs=[flag;posX;posY;posZ;0];
    mode=1;
end

% 10秒后，进入2模式
if mode==1 && t>5
    mode=2;
end


if mode==2
    outCMDs=inCMDs;
end

== matlab function RflyUdpUltraSimpleEight_Dist/Commander13 ==
  data: t input; inCMDs input; outCMDs output
function outCMDs  = fcn(t,inCMDs)

outCMDs=[-1;0;0;0;0]; % 默认空指令，不会发出

persistent mode;

if isempty(mode)
    mode=0;
end


% 进入1阶段，发送起飞指令
if mode==0 && t>1
    flag=11; % 这里对应本地起飞指令
    posX = 200; % x坐标
    posY=0; % y坐标
    posZ=-100;% z坐标
    outCMDs=[flag;posX;posY;posZ;0];
    mode=1;
end

% 10秒后，进入2模式
if mode==1 && t>5
    mode=2;
end


if mode==2
    outCMDs=inCMDs;
end

== matlab function RflyUdpUltraSimpleEight_Dist/Commander1 ==
  data: t input; inCMDs input; outCMDs output
function outCMDs  = fcn(t,inCMDs)

outCMDs=[-1;0;0;0;0]; % 默认空指令，不会发出

persistent mode;

if isempty(mode)
    mode=0;
end


% 进入1阶段，发送起飞指令
if mode==0 && t>3
    flag=11; % 这里对应本地起飞指令
    posX = 500; % x坐标
    posY=0; % y坐标
    posZ=-100;% z坐标
    outCMDs=[flag;posX;posY;posZ;0];
    mode=1;
end

% 10秒后，进入2模式
if mode==1 && t>60
    mode=2;
end


if mode==2
    outCMDs=inCMDs;
end

== matlab function RflyUdpUltraSimpleEight_Dist/Commander ==
  data: t input; inCMDs input; outCMDs output
function outCMDs  = fcn(t,inCMDs)

outCMDs=[-1;0;0;0;0]; % 默认空指令，不会发出

persistent mode;

if isempty(mode)
    mode=0;
end


% 进入1阶段，发送起飞指令
if mode==0 && t>3
    flag=11; % 这里对应本地起飞指令
    posX = 500; % x坐标
    posY=0; % y坐标
    posZ=-100;% z坐标
    outCMDs=[flag;posX;posY;posZ;0];
    mode=1;
end

% 10秒后，进入2模式
if mode==1 && t>60
    mode=2;
end


if mode==2
    outCMDs=inCMDs;
end

== matlab function RflyUdpUltraSimpleEight_Dist/Commander2 ==
  data: t input; inCMDs input; outCMDs output
function outCMDs  = fcn(t,inCMDs)

outCMDs=[-1;0;0;0;0]; % 默认空指令，不会发出

persistent mode;

if isempty(mode)
    mode=0;
end


% 进入1阶段，发送起飞指令
if mode==0 && t>1
    flag=11; % 这里对应本地起飞指令
    posX = 200; % x坐标
    posY=0; % y坐标
    posZ=-100;% z坐标
    outCMDs=[flag;posX;posY;posZ;0];
    mode=1;
end

% 10秒后，进入2模式
if mode==1 && t>5
    mode=2;
end


if mode==2
    outCMDs=inCMDs;
end
